simulink model "RLS_forgetting_factor"  (R2023a)
settings: Solver=FixedStepAuto  StartTime=start_time  StopTime=stop_time  FixedStep=sample_time  RelTol=1e-3
values from neighbouring files (symbols this model uses):
  a = -0.8    [example12.m]    (also in example14.m; example15.m; example16.m)
  b = 0.5    [example12.m]    (also in example14.m; example15.m; example16.m)
  c = -0.5    [example12.m]    (also in example14.m = 0; example15.m = 0; example16.m = 0)
  lambda = Lambda(i)    [example15.m]    (also in example16.m = 0.2)
  mean_e = 0    [example12.m]    (also in example14.m; example15.m)
  P0 = 100 * eye(3)    [example12.m]    (also in example14.m = 0.01 * eye(2); example15.m = 100 * eye(2); example16.m = 0.01)
  sample_time = 1    [example12.m]    (also in example14.m; example15.m; example16.m)
  seed_e = 6    [example12.m]    (also in example14.m = i; example15.m = 2)
  std_e = 0.5    [example12.m]    (also in example14.m; example15.m)
  stop_time = 1000    [example12.m]    (also in example14.m = 20000; example15.m; example16.m)
  theta0 = zeros(3,1)    [example12.m]    (also in example14.m = Theta(:,i); example15.m = zeros(2,1); example16.m = zeros(n_phi, 1))
  y0 = 0    [example14.m]    (also in example15.m)
Description:
  | Example 2_15 Influence of forgetting factor.
settings Model: Creator=Mmoha  LastModifiedBy=Mmoha

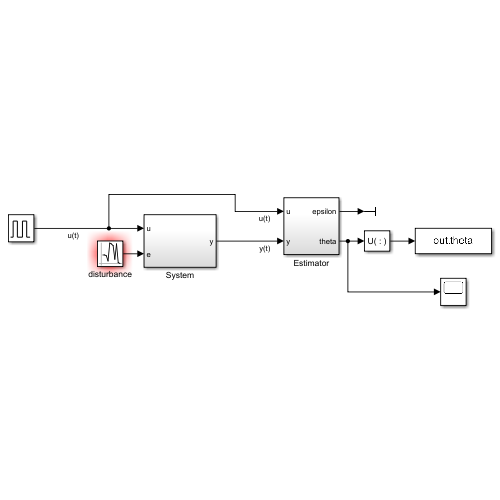
[thumbnail: Simulink's stored preview of the top-level diagram]
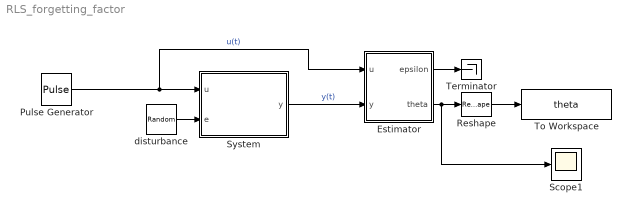
== system RLS_forgetting_factor ==
  Estimator : Subsystem
  Pulse Generator : DiscretePulseGenerator  PulseType=Time based  Period=100  PulseWidth=50
  Reshape : Reshape
  Scope1 : Scope
  System : Subsystem
  Terminator : Terminator
  To Workspace : ToWorkspace  VariableName=theta  SaveFormat=Timeseries  SampleTime=-1
  disturbance : RandomNumber  Mean=mean_e  Variance=std_e^2  Seed=seed_e  SampleTime=sample_time
  wires:
  disturbance/1 -> System/2(e)
  Pulse Generator/1 -> Estimator/1(u), System/1(u)  "u(t)"
  Reshape/1 -> To Workspace/1
  System/1(y) -> Estimator/2(y)  "y(t)"
  Estimator/2(theta) -> Scope1/1, Reshape/1
  Estimator/1(epsilon) -> Terminator/1

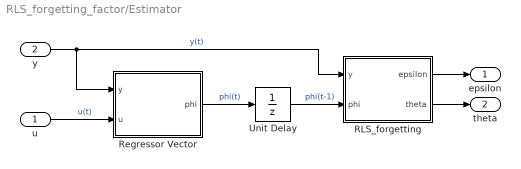
== system RLS_forgetting_factor/Estimator ==
  u : Inport
  y : Inport  Port=2
  RLS_forgetting : Subsystem
  Regressor Vector : Subsystem
  Unit Delay : UnitDelay  SampleTime=-1  HasFrameUpgradeWarning=on
  epsilon : Outport
  theta : Outport  Port=2
  wires:
  u/1 -> Regressor Vector/2(u)  "u(t)"
  Regressor Vector/1(phi) -> Unit Delay/1  "phi(t)"
  y/1 -> Regressor Vector/1(y), RLS_forgetting/1(y)  "y(t)"
  Unit Delay/1 -> RLS_forgetting/2(phi)  "phi(t-1)"
  RLS_forgetting/2(theta) -> theta/1
  RLS_forgetting/1(epsilon) -> epsilon/1

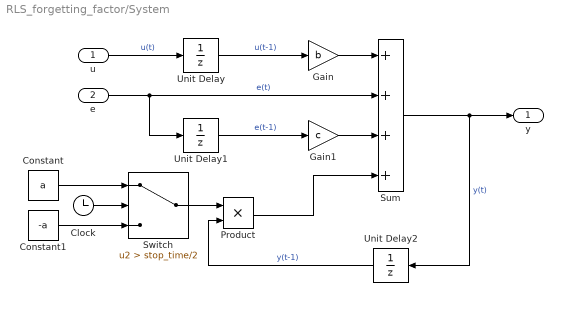
== system RLS_forgetting_factor/System ==
  u : Inport
  e : Inport  Port=2
  Clock : Clock
  Constant : Constant  Value=a
  Constant1 : Constant  Value=-a
  Gain : Gain  Gain=b
  Gain1 : Gain  Gain=c
  Product : Product
  Sum : Sum  Inputs=++++
  Switch : Switch  Criteria=u2 > Threshold  Threshold=stop_time/2  SaturateOnIntegerOverflow=off  InputSameDT=off
  Unit Delay : UnitDelay  SampleTime=-1  HasFrameUpgradeWarning=on
  Unit Delay1 : UnitDelay  SampleTime=-1  HasFrameUpgradeWarning=on
  Unit Delay2 : UnitDelay  InitialCondition=y0  SampleTime=-1  HasFrameUpgradeWarning=on
  y : Outport
  wires:
  u/1 -> Unit Delay/1  "u(t)"
  Unit Delay/1 -> Gain/1  "u(t-1)"
  Gain/1 -> Sum/1
  e/1 -> Unit Delay1/1, Sum/2  "e(t)"
  Unit Delay1/1 -> Gain1/1  "e(t-1)"
  Gain1/1 -> Sum/3
  Sum/1 -> Unit Delay2/1, y/1  "y(t)"
  Product/1 -> Sum/4
  Unit Delay2/1 -> Product/2  "y(t-1)"
  Clock/1 -> Switch/2
  Constant/1 -> Switch/1
  Constant1/1 -> Switch/3
  Switch/1 -> Product/1

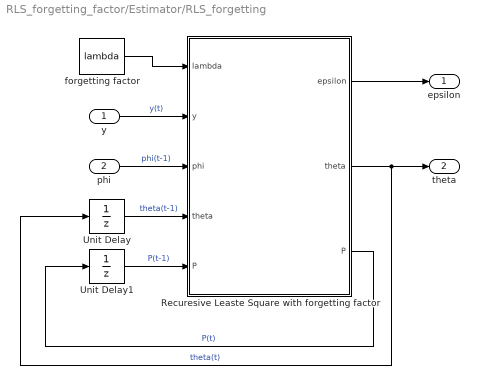
== system RLS_forgetting_factor/Estimator/RLS_forgetting ==
  y : Inport
  phi : Inport  Port=2
  Recuresive Leaste Square with forgetting factor : MATLAB Function  TreatAsAtomicUnit=on
  Unit Delay : UnitDelay  InitialCondition=theta0  SampleTime=-1  HasFrameUpgradeWarning=on
  Unit Delay1 : UnitDelay  InitialCondition=P0  SampleTime=-1  HasFrameUpgradeWarning=on
  forgetting factor : Constant  Value=lambda
  epsilon : Outport
  theta : Outport  Port=2
  wires:
  y/1 -> Recuresive Leaste Square with forgetting factor/2(y)  "y(t)"
  phi/1 -> Recuresive Leaste Square with forgetting factor/3(phi)  "phi(t-1)"
  Unit Delay/1 -> Recuresive Leaste Square with forgetting factor/4("theta ")  "theta(t-1)"
  Unit Delay1/1 -> Recuresive Leaste Square with forgetting factor/5("P ")  "P(t-1)"
  Recuresive Leaste Square with forgetting factor/3(P) -> Unit Delay1/1  "P(t)"
  Recuresive Leaste Square with forgetting factor/2(theta) -> theta/1, Unit Delay/1  "theta(t)"
  Recuresive Leaste Square with forgetting factor/1(epsilon) -> epsilon/1
  forgetting factor/1 -> Recuresive Leaste Square with forgetting factor/1(lambda)

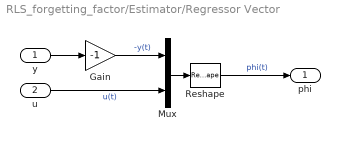
== system RLS_forgetting_factor/Estimator/Regressor Vector ==
  y : Inport
  u : Inport  Port=2
  Gain : Gain  Gain=-1
  Mux : Mux  Inputs=2
  Reshape : Reshape  OutputDimensionality=Column vector (2-D)
  phi : Outport
  wires:
  y/1 -> Gain/1
  Mux/1 -> Reshape/1
  Gain/1 -> Mux/1  "-y(t)"
  u/1 -> Mux/2  "u(t)"
  Reshape/1 -> phi/1  "phi(t)"

== matlab function RLS_forgetting_factor/Estimator/RLS_forgetting/Recuresive Leaste Square with forgetting factor ==
  data: lambda input; y input size=1; epsilon output size=1; phi input size=[2, 1]; theta input size=[2, 1]; P input size=[2, 2]; theta output; P output
function [epsilon, theta, P] = RLS(lambda, y, phi, theta, P)
epsilon = y - phi' * theta;
K = P * phi / (lambda + phi'*P*phi);
P = (eye(2) - K*phi') * P / lambda;
theta = theta + P * phi * epsilon;
